simulink model "iWalkerRoboPeakModel"  (R2014a)
settings: Solver=ode45  StartTime=0.0  StopTime=Inf  RelTol=1e-3
StartFcn:
  | localAddEventListener('iWalkerRoboPeakModel')
libraries: iWalkerLib x3
settings Model: Creator=Brian  LastModifiedBy=Brian
settings OptimizationCC: BlockReduction=off

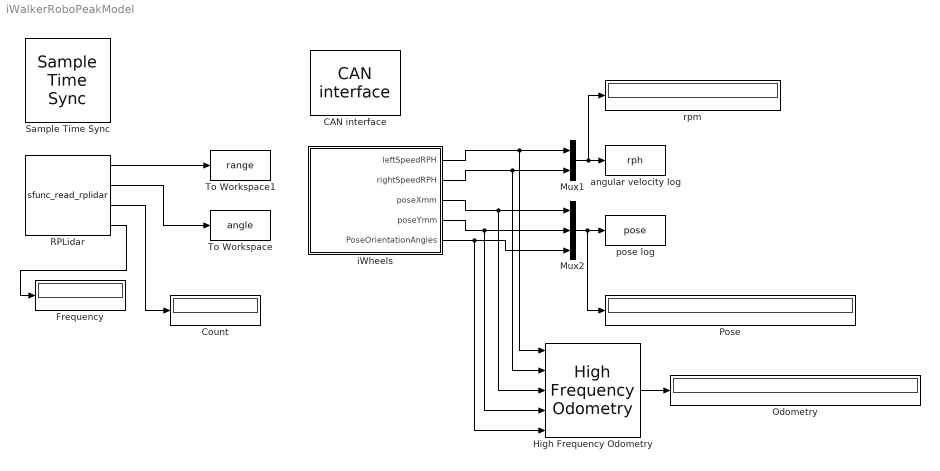
== system iWalkerRoboPeakModel ==
  CAN interface : iWalkerLib/CAN interface
  Count : Display
  Frequency : Display
  High Frequency Odometry : iWalkerLib/High Frequency Odometry
  Mux1 : Mux  Inputs=2
  Mux2 : Mux  Inputs=3
  Odometry : Display
  Pose : Display
  RPLidar : S-Function  FunctionName=sfunc_read_rplidar  EnableBusSupport=off  mask{COM=7, SampleTime=0.3, Verbose=off}
      mask Display:
      | image('rplidar.jpg')
      | port_label('output', 1, 'Range');
      | port_label('output', 2, 'Angle');
      | port_label('output', 3, 'Count');
      | port_label('output', 4, 'Freq');
  Sample Time Sync : iWalkerLib/Sample Time Sync  Priority=8  SampleTime=0.1
  To Workspace : ToWorkspace  VariableName=angle  SaveFormat=Timeseries  SampleTime=-1
  To Workspace1 : ToWorkspace  VariableName=range  SaveFormat=Timeseries  SampleTime=-1
  angular velocity log : ToWorkspace  VariableName=rph  SaveFormat=Timeseries  SampleTime=-1
  iWheels : Subsystem  TreatAsAtomicUnit=on  mask{SampleTime=0.1}
      mask prompts: SampleTime "Sample time"
      mask Display:
      | image('iWheel.jpg')
      | port_label('output', 1, 'left rph')
      | port_label('output', 2, 'right rph')
      | port_label('output', 3, 'x mm')
      | port_label('output', 4, 'y mm')
      | port_label('output', 5, 'theta º')
  pose log : ToWorkspace  VariableName=pose  SaveFormat=Timeseries  SampleTime=-1
  rpm : Display
  wires:
  RPLidar/1 -> To Workspace1/1
  RPLidar/2 -> To Workspace/1
  RPLidar/3 -> Count/1
  RPLidar/4 -> Frequency/1
  Mux1/1 -> rpm/1, angular velocity log/1
  iWheels/1(leftSpeedRPH) -> High Frequency Odometry/1, Mux1/1
  iWheels/2(rightSpeedRPH) -> High Frequency Odometry/2, Mux1/2
  iWheels/3(poseXmm) -> High Frequency Odometry/3, Mux2/1
  iWheels/4(poseYmm) -> High Frequency Odometry/4, Mux2/2
  iWheels/5(PoseOrientationAngles) -> High Frequency Odometry/5, Mux2/3
  Mux2/1 -> Pose/1, pose log/1
  High Frequency Odometry/1 -> Odometry/1

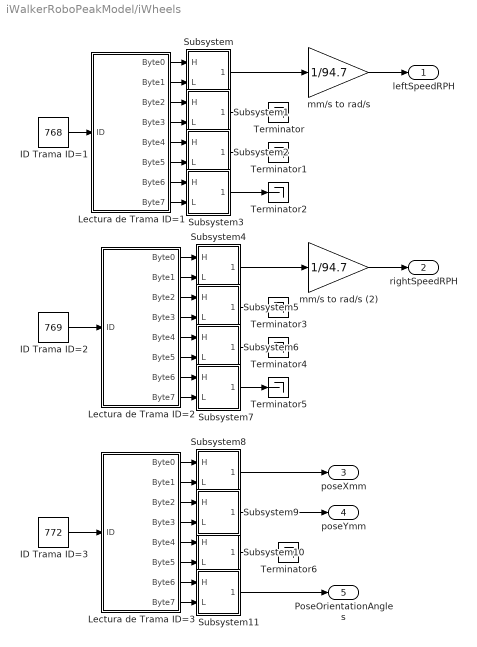
== system iWalkerRoboPeakModel/iWheels ==
  ID Trama ID=1 : Constant  Priority=2  Value=768
  ID Trama ID=2 : Constant  Priority=2  Value=769
  ID Trama ID=3 : Constant  Priority=2  Value=772
  Lectura de Trama ID=1 : Subsystem  Priority=0
  Lectura de Trama ID=2 : Subsystem  Priority=0
  Lectura de Trama ID=3 : Subsystem  Priority=0
  Subsystem : Subsystem
  Subsystem1 : Subsystem
  Subsystem10 : Subsystem
  Subsystem11 : Subsystem
  Subsystem2 : Subsystem
  Subsystem3 : Subsystem
  Subsystem4 : Subsystem
  Subsystem5 : Subsystem
  Subsystem6 : Subsystem
  Subsystem7 : Subsystem
  Subsystem8 : Subsystem
  Subsystem9 : Subsystem
  Terminator{,1..6} (7 alike) : Terminator
  mm/s to rad/s : Gain  Gain=1/94.7
  mm/s to rad/s (2) : Gain  Gain=1/94.7
  leftSpeedRPH : Outport
  rightSpeedRPH : Outport  Port=2
  poseXmm : Outport  Port=3
  poseYmm : Outport  Port=4
  PoseOrientationAngles : Outport  Port=5
  wires:
  ID Trama ID=2/1 -> Lectura de Trama ID=2/1(ID)
  Subsystem7/1(Out1) -> Terminator5/1
  Subsystem6/1(Out1) -> Terminator4/1
  Subsystem5/1(Out1) -> Terminator3/1
  Subsystem4/1(Out1) -> mm/s to rad/s (2)/1
  Subsystem8/1(Out1) -> poseXmm/1
  Subsystem9/1(Out1) -> poseYmm/1
  Subsystem10/1(Out1) -> Terminator6/1
  Subsystem11/1(Out1) -> PoseOrientationAngles/1
  Subsystem3/1(Out1) -> Terminator2/1
  Lectura de Trama ID=1/8(Byte7) -> Subsystem3/2(L)
  Lectura de Trama ID=1/7(Byte6) -> Subsystem3/1(H)
  Subsystem2/1(Out1) -> Terminator1/1
  Lectura de Trama ID=1/6(Byte5) -> Subsystem2/2(L)
  Lectura de Trama ID=1/5(Byte4) -> Subsystem2/1(H)
  Subsystem1/1(Out1) -> Terminator/1
  Lectura de Trama ID=1/4(Byte3) -> Subsystem1/2(L)
  Lectura de Trama ID=1/3(Byte2) -> Subsystem1/1(H)
  Lectura de Trama ID=1/2(Byte1) -> Subsystem/2(L)
  Lectura de Trama ID=1/1(Byte0) -> Subsystem/1(H)
  Subsystem/1(Out1) -> mm/s to rad/s/1
  ID Trama ID=1/1 -> Lectura de Trama ID=1/1(ID)
  Lectura de Trama ID=2/8(Byte7) -> Subsystem7/2(L)
  Lectura de Trama ID=2/7(Byte6) -> Subsystem7/1(H)
  Lectura de Trama ID=2/6(Byte5) -> Subsystem6/2(L)
  Lectura de Trama ID=2/5(Byte4) -> Subsystem6/1(H)
  Lectura de Trama ID=2/4(Byte3) -> Subsystem5/2(L)
  Lectura de Trama ID=2/3(Byte2) -> Subsystem5/1(H)
  Lectura de Trama ID=2/2(Byte1) -> Subsystem4/2(L)
  Lectura de Trama ID=2/1(Byte0) -> Subsystem4/1(H)
  Lectura de Trama ID=3/8(Byte7) -> Subsystem11/2(L)
  Lectura de Trama ID=3/7(Byte6) -> Subsystem11/1(H)
  Lectura de Trama ID=3/6(Byte5) -> Subsystem10/2(L)
  Lectura de Trama ID=3/5(Byte4) -> Subsystem10/1(H)
  Lectura de Trama ID=3/4(Byte3) -> Subsystem9/2(L)
  Lectura de Trama ID=3/3(Byte2) -> Subsystem9/1(H)
  Lectura de Trama ID=3/2(Byte1) -> Subsystem8/2(L)
  Lectura de Trama ID=3/1(Byte0) -> Subsystem8/1(H)
  ID Trama ID=3/1 -> Lectura de Trama ID=3/1(ID)
  mm/s to rad/s (2)/1 -> rightSpeedRPH/1
  mm/s to rad/s/1 -> leftSpeedRPH/1

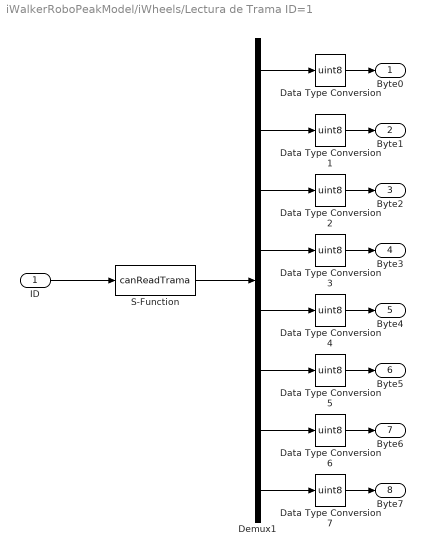
== system iWalkerRoboPeakModel/iWheels/Lectura de Trama ID=1 ==
  ID : Inport
  Data Type Conversion{,1..7} (8 alike) : DataTypeConversion  OutDataTypeStr=uint8  ConvertRealWorld=Stored Integer (SI)
  Demux1 : Demux  Outputs=8
  S-Function : S-Function  Priority=0  FunctionName=canReadTrama  EnableBusSupport=off
  Byte0 : Outport
  Byte1 : Outport  Port=2
  Byte2 : Outport  Port=3
  Byte3 : Outport  Port=4
  Byte4 : Outport  Port=5
  Byte5 : Outport  Port=6
  Byte6 : Outport  Port=7
  Byte7 : Outport  Port=8
  wires:
  ID/1 -> S-Function/1
  S-Function/1 -> Demux1/1
  Data Type Conversion7/1 -> Byte7/1
  Data Type Conversion6/1 -> Byte6/1
  Data Type Conversion5/1 -> Byte5/1
  Data Type Conversion4/1 -> Byte4/1
  Data Type Conversion1/1 -> Byte1/1
  Data Type Conversion/1 -> Byte0/1
  Demux1/1 -> Data Type Conversion/1
  Demux1/2 -> Data Type Conversion1/1
  Demux1/3 -> Data Type Conversion2/1
  Demux1/4 -> Data Type Conversion3/1
  Demux1/5 -> Data Type Conversion4/1
  Demux1/6 -> Data Type Conversion5/1
  Demux1/7 -> Data Type Conversion6/1
  Demux1/8 -> Data Type Conversion7/1
  Data Type Conversion2/1 -> Byte2/1
  Data Type Conversion3/1 -> Byte3/1

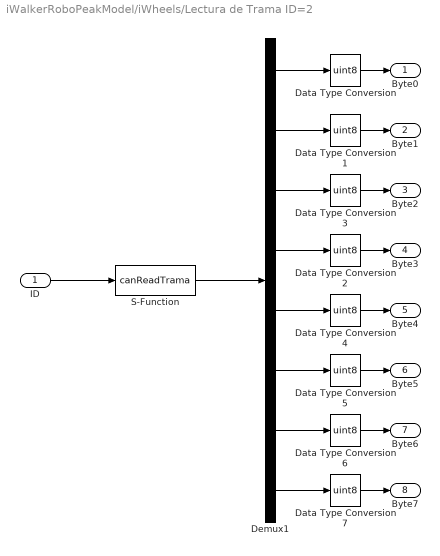
== system iWalkerRoboPeakModel/iWheels/Lectura de Trama ID=2 ==
  ID : Inport
  Data Type Conversion{,1..7} (8 alike) : DataTypeConversion  OutDataTypeStr=uint8  ConvertRealWorld=Stored Integer (SI)
  Demux1 : Demux  Outputs=8
  S-Function : S-Function  Priority=0  FunctionName=canReadTrama  EnableBusSupport=off
  Byte0 : Outport
  Byte1 : Outport  Port=2
  Byte2 : Outport  Port=3
  Byte3 : Outport  Port=4
  Byte4 : Outport  Port=5
  Byte5 : Outport  Port=6
  Byte6 : Outport  Port=7
  Byte7 : Outport  Port=8
  wires:
  Data Type Conversion3/1 -> Byte2/1
  Data Type Conversion2/1 -> Byte3/1
  ID/1 -> S-Function/1
  S-Function/1 -> Demux1/1
  Data Type Conversion7/1 -> Byte7/1
  Data Type Conversion6/1 -> Byte6/1
  Data Type Conversion5/1 -> Byte5/1
  Data Type Conversion4/1 -> Byte4/1
  Data Type Conversion1/1 -> Byte1/1
  Data Type Conversion/1 -> Byte0/1
  Demux1/1 -> Data Type Conversion/1
  Demux1/2 -> Data Type Conversion1/1
  Demux1/3 -> Data Type Conversion3/1
  Demux1/4 -> Data Type Conversion2/1
  Demux1/5 -> Data Type Conversion4/1
  Demux1/6 -> Data Type Conversion5/1
  Demux1/7 -> Data Type Conversion6/1
  Demux1/8 -> Data Type Conversion7/1

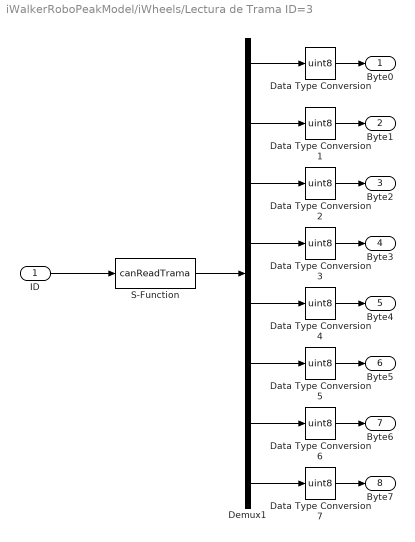
== system iWalkerRoboPeakModel/iWheels/Lectura de Trama ID=3 ==
  ID : Inport
  Data Type Conversion{,1..7} (8 alike) : DataTypeConversion  OutDataTypeStr=uint8  ConvertRealWorld=Stored Integer (SI)
  Demux1 : Demux  Outputs=8
  S-Function : S-Function  Priority=0  FunctionName=canReadTrama  EnableBusSupport=off
  Byte0 : Outport
  Byte1 : Outport  Port=2
  Byte2 : Outport  Port=3
  Byte3 : Outport  Port=4
  Byte4 : Outport  Port=5
  Byte5 : Outport  Port=6
  Byte6 : Outport  Port=7
  Byte7 : Outport  Port=8
  wires:
  ID/1 -> S-Function/1
  S-Function/1 -> Demux1/1
  Data Type Conversion7/1 -> Byte7/1
  Data Type Conversion6/1 -> Byte6/1
  Data Type Conversion5/1 -> Byte5/1
  Data Type Conversion4/1 -> Byte4/1
  Data Type Conversion1/1 -> Byte1/1
  Data Type Conversion/1 -> Byte0/1
  Demux1/1 -> Data Type Conversion/1
  Demux1/2 -> Data Type Conversion1/1
  Demux1/3 -> Data Type Conversion2/1
  Demux1/4 -> Data Type Conversion3/1
  Demux1/5 -> Data Type Conversion4/1
  Demux1/6 -> Data Type Conversion5/1
  Demux1/7 -> Data Type Conversion6/1
  Demux1/8 -> Data Type Conversion7/1
  Data Type Conversion2/1 -> Byte2/1
  Data Type Conversion3/1 -> Byte3/1

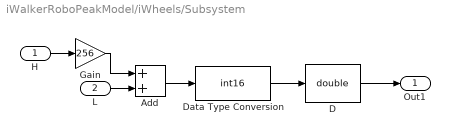
== system iWalkerRoboPeakModel/iWheels/Subsystem ==
  H : Inport
  L : Inport  Port=2
  Add : Sum
  D : DataTypeConversion  OutDataTypeStr=double  ConvertRealWorld=Stored Integer (SI)
  Data Type Conversion : DataTypeConversion  OutDataTypeStr=int16
  Gain : Gain  Gain=256
  Out1 : Outport
  wires:
  Gain/1 -> Add/1
  H/1 -> Gain/1
  L/1 -> Add/2
  Add/1 -> Data Type Conversion/1
  Data Type Conversion/1 -> D/1
  D/1 -> Out1/1

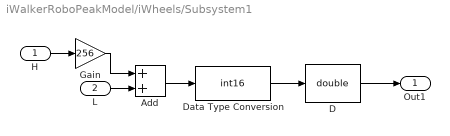
== system iWalkerRoboPeakModel/iWheels/Subsystem1 ==
  H : Inport
  L : Inport  Port=2
  Add : Sum
  D : DataTypeConversion  OutDataTypeStr=double  ConvertRealWorld=Stored Integer (SI)
  Data Type Conversion : DataTypeConversion  OutDataTypeStr=int16
  Gain : Gain  Gain=256
  Out1 : Outport
  wires:
  D/1 -> Out1/1
  Data Type Conversion/1 -> D/1
  Add/1 -> Data Type Conversion/1
  L/1 -> Add/2
  H/1 -> Gain/1
  Gain/1 -> Add/1

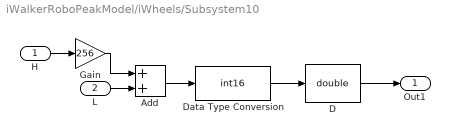
== system iWalkerRoboPeakModel/iWheels/Subsystem10 ==
  H : Inport
  L : Inport  Port=2
  Add : Sum
  D : DataTypeConversion  OutDataTypeStr=double  ConvertRealWorld=Stored Integer (SI)
  Data Type Conversion : DataTypeConversion  OutDataTypeStr=int16
  Gain : Gain  Gain=256
  Out1 : Outport
  wires:
  Gain/1 -> Add/1
  H/1 -> Gain/1
  L/1 -> Add/2
  Add/1 -> Data Type Conversion/1
  Data Type Conversion/1 -> D/1
  D/1 -> Out1/1

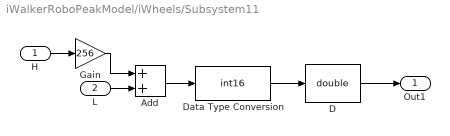
== system iWalkerRoboPeakModel/iWheels/Subsystem11 ==
  H : Inport
  L : Inport  Port=2
  Add : Sum
  D : DataTypeConversion  OutDataTypeStr=double  ConvertRealWorld=Stored Integer (SI)
  Data Type Conversion : DataTypeConversion  OutDataTypeStr=int16
  Gain : Gain  Gain=256
  Out1 : Outport
  wires:
  D/1 -> Out1/1
  Data Type Conversion/1 -> D/1
  Add/1 -> Data Type Conversion/1
  L/1 -> Add/2
  H/1 -> Gain/1
  Gain/1 -> Add/1

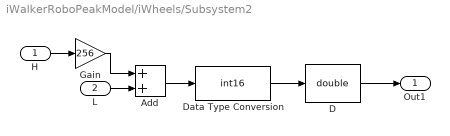
== system iWalkerRoboPeakModel/iWheels/Subsystem2 ==
  H : Inport
  L : Inport  Port=2
  Add : Sum
  D : DataTypeConversion  OutDataTypeStr=double  ConvertRealWorld=Stored Integer (SI)
  Data Type Conversion : DataTypeConversion  OutDataTypeStr=int16
  Gain : Gain  Gain=256
  Out1 : Outport
  wires:
  Gain/1 -> Add/1
  H/1 -> Gain/1
  L/1 -> Add/2
  Add/1 -> Data Type Conversion/1
  Data Type Conversion/1 -> D/1
  D/1 -> Out1/1

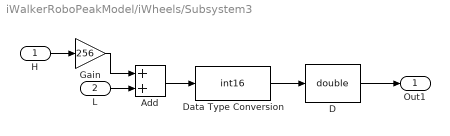
== system iWalkerRoboPeakModel/iWheels/Subsystem3 ==
  H : Inport
  L : Inport  Port=2
  Add : Sum
  D : DataTypeConversion  OutDataTypeStr=double  ConvertRealWorld=Stored Integer (SI)
  Data Type Conversion : DataTypeConversion  OutDataTypeStr=int16
  Gain : Gain  Gain=256
  Out1 : Outport
  wires:
  D/1 -> Out1/1
  Data Type Conversion/1 -> D/1
  Add/1 -> Data Type Conversion/1
  L/1 -> Add/2
  H/1 -> Gain/1
  Gain/1 -> Add/1

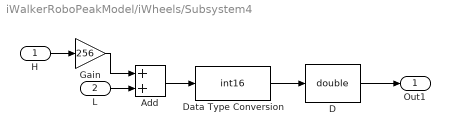
== system iWalkerRoboPeakModel/iWheels/Subsystem4 ==
  H : Inport
  L : Inport  Port=2
  Add : Sum
  D : DataTypeConversion  OutDataTypeStr=double  ConvertRealWorld=Stored Integer (SI)
  Data Type Conversion : DataTypeConversion  OutDataTypeStr=int16
  Gain : Gain  Gain=256
  Out1 : Outport
  wires:
  Gain/1 -> Add/1
  H/1 -> Gain/1
  L/1 -> Add/2
  Add/1 -> Data Type Conversion/1
  Data Type Conversion/1 -> D/1
  D/1 -> Out1/1

== system iWalkerRoboPeakModel/iWheels/Subsystem5 ==
  H : Inport
  L : Inport  Port=2
  Add : Sum
  D : DataTypeConversion  OutDataTypeStr=double  ConvertRealWorld=Stored Integer (SI)
  Data Type Conversion : DataTypeConversion  OutDataTypeStr=int16
  Gain : Gain  Gain=256
  Out1 : Outport
  wires:
  D/1 -> Out1/1
  Data Type Conversion/1 -> D/1
  Add/1 -> Data Type Conversion/1
  L/1 -> Add/2
  H/1 -> Gain/1
  Gain/1 -> Add/1

== system iWalkerRoboPeakModel/iWheels/Subsystem6 ==
  H : Inport
  L : Inport  Port=2
  Add : Sum
  D : DataTypeConversion  OutDataTypeStr=double  ConvertRealWorld=Stored Integer (SI)
  Data Type Conversion : DataTypeConversion  OutDataTypeStr=int16
  Gain : Gain  Gain=256
  Out1 : Outport
  wires:
  Gain/1 -> Add/1
  H/1 -> Gain/1
  L/1 -> Add/2
  Add/1 -> Data Type Conversion/1
  Data Type Conversion/1 -> D/1
  D/1 -> Out1/1

== system iWalkerRoboPeakModel/iWheels/Subsystem7 ==
  H : Inport
  L : Inport  Port=2
  Add : Sum
  D : DataTypeConversion  OutDataTypeStr=double  ConvertRealWorld=Stored Integer (SI)
  Data Type Conversion : DataTypeConversion  OutDataTypeStr=int16
  Gain : Gain  Gain=256
  Out1 : Outport
  wires:
  D/1 -> Out1/1
  Data Type Conversion/1 -> D/1
  Add/1 -> Data Type Conversion/1
  L/1 -> Add/2
  H/1 -> Gain/1
  Gain/1 -> Add/1

== system iWalkerRoboPeakModel/iWheels/Subsystem8 ==
  H : Inport
  L : Inport  Port=2
  Add : Sum
  D : DataTypeConversion  OutDataTypeStr=double  ConvertRealWorld=Stored Integer (SI)
  Data Type Conversion : DataTypeConversion  OutDataTypeStr=int16
  Gain : Gain  Gain=256
  Out1 : Outport
  wires:
  Gain/1 -> Add/1
  H/1 -> Gain/1
  L/1 -> Add/2
  Add/1 -> Data Type Conversion/1
  Data Type Conversion/1 -> D/1
  D/1 -> Out1/1

== system iWalkerRoboPeakModel/iWheels/Subsystem9 ==
  H : Inport
  L : Inport  Port=2
  Add : Sum
  D : DataTypeConversion  OutDataTypeStr=double  ConvertRealWorld=Stored Integer (SI)
  Data Type Conversion : DataTypeConversion  OutDataTypeStr=int16
  Gain : Gain  Gain=256
  Out1 : Outport
  wires:
  D/1 -> Out1/1
  Data Type Conversion/1 -> D/1
  Add/1 -> Data Type Conversion/1
  L/1 -> Add/2
  H/1 -> Gain/1
  Gain/1 -> Add/1
